simulink model "IEEE_3CIG_9bus_sapc"  (R2024a)
settings: Solver=ode8  StartTime=0.0  StopTime=110  RelTol=1e-4  EnableMultiTasking=on
PreLoadFcn:
  | ct = 1.083
undefined symbols (not defined in the file): D1, Delta, kp1, kp2, kp3, Pmax1, Pmax2, Pmax3, Pmin1, Pmin2, Pmin3, ts_pi
libraries: spsThreePhaseVIMeasurementLib x12, spsLoadFlowBusLib x9, spsPLL3phLib x9, spsSequenceAnalyzerLib x9, eeSinusoidalMeasurementV2 x9, spsThreePhasePISectionLineLib x6, jailib x5, spsThreePhaseTransformerTwoWindingsLib x3, spsDCVoltageSourceLib x3, spsMeanLib x3, spsUniversalBridgeLib x3, slpidlib x2
(part 2 of 2)

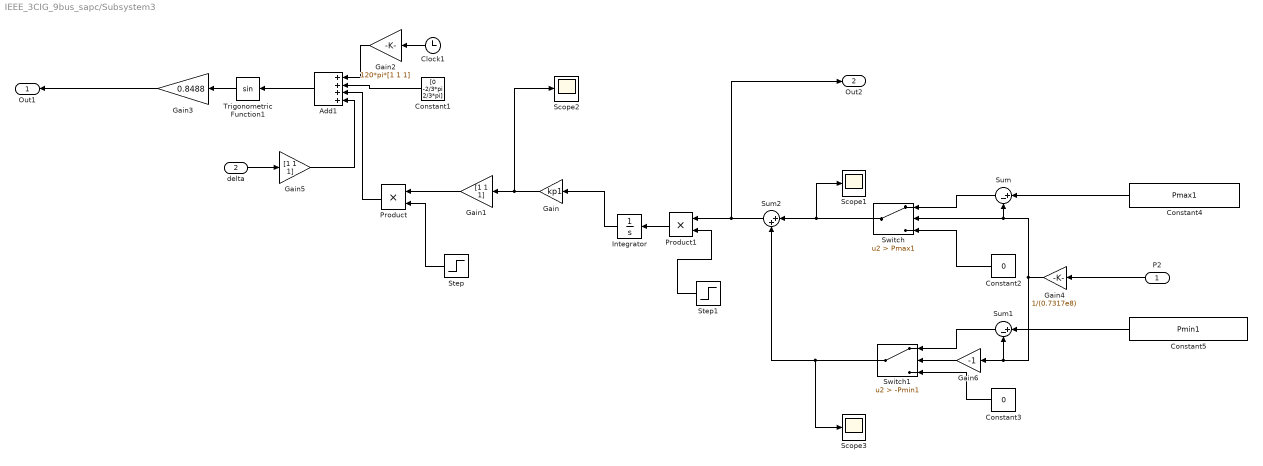
== system IEEE_3CIG_9bus_sapc/Subsystem3 ==
  P2 : Inport
  delta : Inport  Port=2
  Add1 : Sum  Inputs=++++
  Clock1 : Clock
  Constant1 : Constant  Value="[0  -2/3*pi   2/3*pi]"
  Constant2 : Constant  Value=0
  Constant3 : Constant  Value=0
  Constant4 : Constant  Value=Pmax1
  Constant5 : Constant  Value=Pmin1
  Gain : Gain  Gain=kp1
  Gain1 : Gain  Gain=[1 1 1]
  Gain2 : Gain  Gain=120*pi*[1 1 1]
  Gain3 : Gain  Gain=0.8488
  Gain4 : Gain  Gain=1/(0.7317e8)
  Gain5 : Gain  Gain=[1 1 1]
  Gain6 : Gain  Gain=-1
  Integrator : Integrator
  Product : Product
  Product1 : Product
  Scope1 : Scope
  Scope2 : Scope
  Scope3 : Scope
  Step : Step  Time=5  SampleTime=0
  Step1 : Step  Time=5  SampleTime=0
  Sum : Sum  Inputs=|+-
  Sum1 : Sum  Inputs=|+-
  Sum2 : Sum  Inputs=|++
  Switch : Switch  Criteria=u2 > Threshold  Threshold=Pmax1  SaturateOnIntegerOverflow=off  InputSameDT=off
  Switch1 : Switch  Criteria=u2 > Threshold  Threshold=-Pmin1  SaturateOnIntegerOverflow=off  InputSameDT=off
  Trigonometric Function1 : Trigonometry
  Out1 : Outport
  Out2 : Outport  Port=2
  wires:
  Clock1/1 -> Gain2/1
  Constant1/1 -> Add1/2
  Gain2/1 -> Add1/1
  Add1/1 -> Trigonometric Function1/1
  Gain1/1 -> Product/1
  Step/1 -> Product/2
  Product/1 -> Add1/3
  Trigonometric Function1/1 -> Gain3/1
  Gain3/1 -> Out1/1
  Gain/1 -> Scope2/1, Gain1/1
  Integrator/1 -> Gain/1
  P2/1 -> Gain4/1
  delta/1 -> Gain5/1
  Gain5/1 -> Add1/4
  Step1/1 -> Product1/2
  Product1/1 -> Integrator/1
  Constant4/1 -> Sum/1
  Sum/1 -> Switch/1
  Constant2/1 -> Switch/3
  Constant5/1 -> Sum1/1
  Sum1/1 -> Switch1/1
  Gain4/1 -> Gain6/1, Sum1/2, Sum/2, Switch/2
  Constant3/1 -> Switch1/3
  Gain6/1 -> Switch1/2
  Switch/1 -> Scope1/1, Sum2/1
  Switch1/1 -> Scope3/1, Sum2/2
  Sum2/1 -> Out2/1, Product1/1
